simulink library "ovenLib"  (R2016a)
settings: Solver=ode45  StartTime=0.0  StopTime=10.0  RelTol=1e-3
undefined symbols (not defined in the file): des, N
libraries: fl_lib x33, simulink x18, nesl_utility x11, PJPhysLib_lib x3
(part 2 of 2)

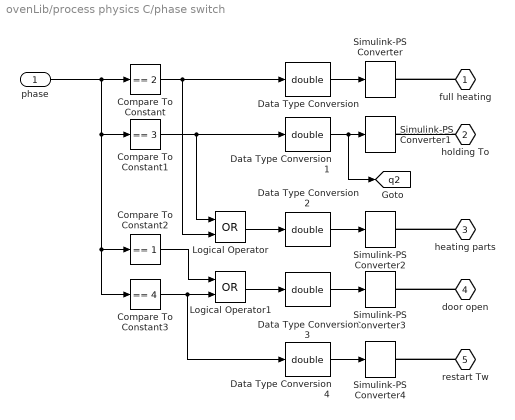
== system ovenLib/process physics C/phase switch ==
  phase : Inport
  Compare To Constant : simulink/Logic and Bit Operations/Compare To Constant  relop===  const=2  OutDataTypeStr=boolean
  Compare To Constant1 : simulink/Logic and Bit Operations/Compare To Constant  relop===  const=3  OutDataTypeStr=boolean
  Compare To Constant2 : simulink/Logic and Bit Operations/Compare To Constant  relop===  const=1  OutDataTypeStr=boolean
  Compare To Constant3 : simulink/Logic and Bit Operations/Compare To Constant  relop===  const=4  OutDataTypeStr=boolean
  Data Type Conversion{,1..4} (5 alike) : DataTypeConversion  OutDataTypeStr=double
  Logical Operator : Logic  Operator=OR  AllPortsSameDT=off  OutDataTypeStr=boolean
  Logical Operator1 : Logic  Operator=OR  AllPortsSameDT=off  OutDataTypeStr=boolean
  Simulink-PS Converter{,1..4} (5 alike) : nesl_utility/Simulink-PS Converter  PhysicalDomain=network_engine_domain  SubClassName=ps_input  LeftPortType=input  RightPortType=output  PseudoPeriodic=off  Frequencies=[]  NoiseDistribution=none  NoiseParameters=[]  Unit=1  AffineConversion=off  InputFiltering=off  SimscapeFilterOrder=1  InputFilterTimeConstant=0.001  UdotUserProvided=1
  full heating : PMIOPort  Port=1  Side=Right
  holding To : PMIOPort  Port=2  Side=Right
  heating parts : PMIOPort  Port=3  Side=Right
  door open : PMIOPort  Port=4  Side=Right
  restart Tw : PMIOPort  Port=5  Side=Right
  tag scope: q2=global
  wires:
  Data Type Conversion4/1 -> Simulink-PS Converter4/1
  Data Type Conversion3/1 -> Simulink-PS Converter3/1
  Data Type Conversion2/1 -> Simulink-PS Converter2/1
  Data Type Conversion1/1 -> Simulink-PS Converter1/1, [q2]
  Data Type Conversion/1 -> Simulink-PS Converter/1
  Compare To Constant2/1 -> Logical Operator1/1
  Compare To Constant3/1 -> Logical Operator1/2, Data Type Conversion4/1
  Logical Operator1/1 -> Data Type Conversion3/1
  Logical Operator/1 -> Data Type Conversion2/1
  Compare To Constant1/1 -> Data Type Conversion1/1, Logical Operator/1
  Compare To Constant/1 -> Data Type Conversion/1, Logical Operator/2
  phase/1 -> Compare To Constant/1, Compare To Constant1/1, Compare To Constant2/1, Compare To Constant3/1
  connections:
  restart Tw/RConn1 -- Simulink-PS Converter4/RConn1
  door open/RConn1 -- Simulink-PS Converter3/RConn1
  heating parts/RConn1 -- Simulink-PS Converter2/RConn1
  holding To/RConn1 -- Simulink-PS Converter1/RConn1
  full heating/RConn1 -- Simulink-PS Converter/RConn1

== system ovenLib/source/Attribute Function ==
  MATLAB Function : MATLAB Function  TreatAsAtomicUnit=on
  __DMLF__EDE2FCE__ : EntityDepartureFunctionCallGenerator  TimingFunctionCallF1=Before entity departure  IsInsideAFB=on
  __DMLF__GA__ : GetAttribute  AttributeName=part_no|nr_wp  AttributeMissing=Error|Error  AttributeDefaultValue=1|1  AttributeTreatAsVector=1|1  AttributeSendTiming=Before entity departure|Before entity departure  EvaluatedDefaultAttributeValue={ [];[]}  IsInsideAFB=on
      settings: OutputPortMap=o1,o2
  __DMLF__SA__ : SetAttribute  AttributeName=port  AttributeFrom=Signal port  EvaluatedAttributeValue={ []}  IsInsideAFB=on
  IN : PMIOPort  Port=1  Side=Left
  OUT : PMIOPort  Port=2  Side=Right
  wires:
  MATLAB Function/1(out_port) -> __DMLF__SA__/1
  __DMLF__GA__/2 -> MATLAB Function/2(nr_wp)
  __DMLF__GA__/1 -> MATLAB Function/1(part_no)
  __DMLF__EDE2FCE__/1 -> MATLAB Function/Trigger
  connections:
  __DMLF__SA__/LConn1 -- __DMLF__EDE2FCE__/RConn1
  __DMLF__GA__/RConn1 -- __DMLF__EDE2FCE__/LConn1
  IN/RConn1 -- __DMLF__GA__/LConn1
  __DMLF__SA__/RConn1 -- OUT/RConn1

== system ovenLib/process control A/phase 2 heatUp/Choose path ==
  To : Inport
  Bias : Bias  Bias=1
  Data Type Conversion : DataTypeConversion  OutDataTypeStr=double
  Relational Operator : RelationalOperator  Operator=<=  OutDataTypeStr=boolean
  Ts : Constant  Value=Tset
  path : Outport
  wires:
  Data Type Conversion/1 -> Bias/1
  To/1 -> Relational Operator/2
  Relational Operator/1 -> Data Type Conversion/1
  Bias/1 -> path/1
  Ts/1 -> Relational Operator/1

== system ovenLib/process control B/Phase 2 heatUp/Choose path ==
  Tsoll : Inport
  To : Inport  Port=2
  Bias : Bias  Bias=1
  Data Type Conversion : DataTypeConversion  OutDataTypeStr=double
  Relational Operator : RelationalOperator  Operator=<=  OutDataTypeStr=boolean
  path : Outport
  wires:
  To/1 -> Relational Operator/2
  Bias/1 -> path/1
  Tsoll/1 -> Relational Operator/1
  Data Type Conversion/1 -> Bias/1
  Relational Operator/1 -> Data Type Conversion/1

== system ovenLib/process control B/Phase 2 heatUp/setHeatPValues ==
  MATLAB Function : MATLAB Function  TreatAsAtomicUnit=on
  __DMLF__EDE2FCE__ : EntityDepartureFunctionCallGenerator  TimingFunctionCallF1=Before entity departure  IsInsideAFB=on
  __DMLF__GA__ : GetAttribute  AttributeName=nextHeatPNo|HeatP  AttributeMissing=Error|Error  AttributeDefaultValue=1|1  AttributeTreatAsVector=1|1  AttributeSendTiming=Before entity departure|Before entity departure  EvaluatedDefaultAttributeValue={ [];[]}  IsInsideAFB=on
      settings: OutputPortMap=o1,o2
  __DMLF__SA__ : SetAttribute  AttributeName=HeatPTemp|HeatPTime  AttributeFrom=Signal port|Signal port  AttributeValue=1|1  AttributeTreatAsVector=1|1  EvaluatedAttributeValue={ [];[]}  IsInsideAFB=on
      settings: InputPortMap=u0,u1
  IN : PMIOPort  Port=1  Side=Left
  OUT : PMIOPort  Port=2  Side=Right
  wires:
  __DMLF__EDE2FCE__/1 -> MATLAB Function/Trigger
  __DMLF__GA__/1 -> MATLAB Function/1(nextHeatPNo)
  __DMLF__GA__/2 -> MATLAB Function/2(HeatP)
  MATLAB Function/1(out_HeatPTemp) -> __DMLF__SA__/1
  MATLAB Function/2(out_HeatPTime) -> __DMLF__SA__/2
  connections:
  __DMLF__SA__/RConn1 -- OUT/RConn1
  IN/RConn1 -- __DMLF__GA__/LConn1
  __DMLF__GA__/RConn1 -- __DMLF__EDE2FCE__/LConn1
  __DMLF__SA__/LConn1 -- __DMLF__EDE2FCE__/RConn1

== system ovenLib/process control B/Phase 3 hold/Set Out Port ==
  MATLAB Function : MATLAB Function  TreatAsAtomicUnit=on
  __DMLF__EDE2FCE__ : EntityDepartureFunctionCallGenerator  TimingFunctionCallF1=Before entity departure  IsInsideAFB=on
  __DMLF__GA__ : GetAttribute  AttributeName=nextHeatPNo|HeatP  AttributeMissing=Error|Error  AttributeDefaultValue=1|1  AttributeTreatAsVector=1|1  AttributeSendTiming=Before entity departure|Before entity departure  EvaluatedDefaultAttributeValue={ [];[]}  IsInsideAFB=on
      settings: OutputPortMap=o1,o2
  __DMLF__SA__ : SetAttribute  AttributeName=nextHeatPNo|OutPort  AttributeFrom=Signal port|Signal port  AttributeValue=1|1  AttributeTreatAsVector=1|1  EvaluatedAttributeValue={ [];[]}  IsInsideAFB=on
      settings: InputPortMap=u0,u1
  IN : PMIOPort  Port=1  Side=Left
  OUT : PMIOPort  Port=2  Side=Right
  wires:
  __DMLF__EDE2FCE__/1 -> MATLAB Function/Trigger
  __DMLF__GA__/1 -> MATLAB Function/1(nextHeatPNo)
  __DMLF__GA__/2 -> MATLAB Function/2(HeatP)
  MATLAB Function/1(out_nextHeatPNo) -> __DMLF__SA__/1
  MATLAB Function/2(out_OutPort) -> __DMLF__SA__/2
  connections:
  __DMLF__SA__/RConn1 -- OUT/RConn1
  IN/RConn1 -- __DMLF__GA__/LConn1
  __DMLF__GA__/RConn1 -- __DMLF__EDE2FCE__/LConn1
  __DMLF__SA__/LConn1 -- __DMLF__EDE2FCE__/RConn1

== system ovenLib/process physics C/Set T/Tfix ==
  Conductive Heat Transfer10 : fl_lib/Thermal/Thermal Elements/Conductive Heat Transfer  area=10 m^2  thickness=1 m  th_cond=10000 W/(m*K)  Q_specify=off  Q_priority=High  Q=0 J/s  T_specify=off  T_priority=High  T=0 K
  Ideal Temperature Source : fl_lib/Thermal/Thermal Sources/Ideal Temperature Source
  Thermal Reference : fl_lib/Thermal/Thermal Elements/Thermal Reference
  T : PMIOPort  Port=1  Side=Left
  Port : PMIOPort  Port=2  Side=Right
  connections:
  T/RConn1 -- Ideal Temperature Source/RConn1
  Conductive Heat Transfer10/LConn1 -- Port/RConn1
  Thermal Reference/LConn1 -- Ideal Temperature Source/RConn2
  Ideal Temperature Source/LConn1 -- Conductive Heat Transfer10/RConn1

== system ovenLib/process physics C/T measurement/T sensor 1 ==
  Ideal Temperature Sensor1 : fl_lib/Thermal/Thermal Sensors/Ideal Temperature Sensor
  PS-Simulink Converter : nesl_utility/PS-Simulink Converter  PhysicalDomain=network_engine_domain  SubClassName=ps_output  LeftPortType=input  RightPortType=output  PseudoPeriodic=off  Frequencies=[]  Unit=1  AffineConversion=off
  Thermal Reference1 : fl_lib/Thermal/Thermal Elements/Thermal Reference
  Port : PMIOPort  Port=1  Side=Left
  T : Outport
  wires:
  PS-Simulink Converter/1 -> T/1
  connections:
  Ideal Temperature Sensor1/RConn2 -- PS-Simulink Converter/LConn1
  Ideal Temperature Sensor1/LConn1 -- Port/RConn1
  Ideal Temperature Sensor1/RConn1 -- Thermal Reference1/LConn1

== system ovenLib/process physics C/T measurement/T sensor 2 ==
  Ideal Temperature Sensor1 : fl_lib/Thermal/Thermal Sensors/Ideal Temperature Sensor
  PS-Simulink Converter : nesl_utility/PS-Simulink Converter  PhysicalDomain=network_engine_domain  SubClassName=ps_output  LeftPortType=input  RightPortType=output  PseudoPeriodic=off  Frequencies=[]  Unit=1  AffineConversion=off
  Thermal Reference1 : fl_lib/Thermal/Thermal Elements/Thermal Reference
  Port : PMIOPort  Port=1  Side=Left
  T : Outport
  wires:
  PS-Simulink Converter/1 -> T/1
  connections:
  Ideal Temperature Sensor1/RConn1 -- Thermal Reference1/LConn1
  Ideal Temperature Sensor1/LConn1 -- Port/RConn1
  Ideal Temperature Sensor1/RConn2 -- PS-Simulink Converter/LConn1

== matlab function ovenLib/source/Attribute Function/MATLAB Function ==
  data: part_no input; out_port output; nr_wp input
  events: trigger input FUNCTION_CALL_EVENT
function out_port  = fcn(part_no,nr_wp)
%FCN    Access and modify attributes with Embedded MATLAB Function 
% 
% Input arguments must match the attribute names.
% Output arguments must be out_<AttributeName>,
% e.g., out_ServiceTime where ServiceTime is the attribute name.
% 
% The output attribute will be created if it is not present.
%
if part_no<=nr_wp
    out_port = 1;
else
    out_port = 2;
end

== stateflow chart ovenLib/process control C/DEVS ==
  settings: executeAtInitialization=1
  state ProcDEVS [parallel]
    settings: executionOrder=1
    state loading
      en: phase = 1;
      sigma = 5*60; newSigma;
    state wait
      en: sH = ml.size(HeatP,1);
    state heatUp
      en: phase= 2;Tset = HeatP[idxT+1][2];
      ex: idxDt++;idxT = idxT+2;
    state checkT
      en: Tset = HeatP[2][2];
      sigma = 1; newSigma;
    state hold
      en: phase =3;
      sigma = (HeatP[idxDt+1][1]- HeatP[idxDt][1])*60;
      newSigma;
      ex: idxDt++;
    state unload
      en: phase = 4;
      sigma = 5*60; newSigma;
    state coolDown
      en: phase = 5;
    (default) -> wait
    coolDown -> wait [order 2] : coolDownReady{phase = 0;}
    wait -> loading : after(max_capa,entityIn)
    coolDown -> loading [order 1] : after(max_capa,entityIn)
    loading -> checkT : DEVS{idxT=1;idxDt=1;}
    checkT -> heatUp [order 2]
    hold -> heatUp [order 2] : DEVS[idxT<sH]
    heatUp -> hold : heatUpReady
    checkT -> hold [order 1] : heatUpReady
        | {idxDt++;idxT = idxT+2;}
    hold -> unload [order 1] : DEVS[idxT==sH]
    unload -> coolDown : DEVS{send(oG,GateControl)}
  state GateControl [parallel]
    settings: executionOrder=2
    state closed
    state open
      en:openGate;
      i++; sigma = 0;
      newSigma;
    (default) -> closed
    open -> closed [order 1] : [i==max_capa]/i=0;
    closed -> open : oG
    open -> open [order 2]
  data: sigma output double; Tset output double; max_capa input double; i local double =0; HeatP input; idxT local double =1; idxDt local double =1; sH local double; phase output double
  events: entityIn input FUNCTION_CALL_EVENT; oG local FUNCTION_CALL_EVENT; DEVS input FUNCTION_CALL_EVENT; newSigma output FUNCTION_CALL_EVENT; openGate output FUNCTION_CALL_EVENT; heatUpReady input FUNCTION_CALL_EVENT; coolDownReady input FUNCTION_CALL_EVENT

== matlab function ovenLib/process control B/Phase 2 heatUp/setHeatPValues/MATLAB Function ==
  data: nextHeatPNo input; out_HeatPTemp output; out_HeatPTime output; HeatP input
  events: trigger input FUNCTION_CALL_EVENT
function [out_HeatPTemp, out_HeatPTime] = fcn(nextHeatPNo, HeatP)
%FCN    Access and modify attributes with MATLAB 
% 
% Input arguments must match the attribute names.
% Output arguments must be out_<AttributeName>,
% e.g., out_ServiceTime where ServiceTime is the attribute name.
% 
% The output attribute will be created if it is not present.
%

out_HeatPTime = 60*HeatP(nextHeatPNo, 1);
out_HeatPTemp = HeatP(nextHeatPNo, 2);

== matlab function ovenLib/process control B/Phase 3 hold/Set Out Port/MATLAB Function ==
  data: nextHeatPNo input; out_nextHeatPNo output; out_OutPort output; HeatP input
  events: trigger input FUNCTION_CALL_EVENT
function [out_nextHeatPNo, out_OutPort] = fcn(nextHeatPNo, HeatP)
%FCN    Access and modify attributes with MATLAB 
% 
% Input arguments must match the attribute names.
% Output arguments must be out_<AttributeName>,
% e.g., out_ServiceTime where ServiceTime is the attribute name.
% 
% The output attribute will be created if it is not present.
%

out_nextHeatPNo = nextHeatPNo + 1;
if out_nextHeatPNo > size(HeatP,1) 
  out_OutPort = 1;
else
  out_OutPort = 2;
end
